simulink model "ensaios"  (R2012b)
settings: Solver=ode3  StartTime=0.0  StopTime=2  FixedStep=1e-4  RelTol=1e-6
libraries: BLDC x1
settings Model: BufferReuse=off  Creator=Juliano  LastModifiedBy=Juliano
settings DataIOCC: LimitDataPoints=off
settings OptimizationCC: OptimizeBlockIOStorage=off  BufferReuse=off  ExpressionFolding=off  LocalBlockOutputs=off

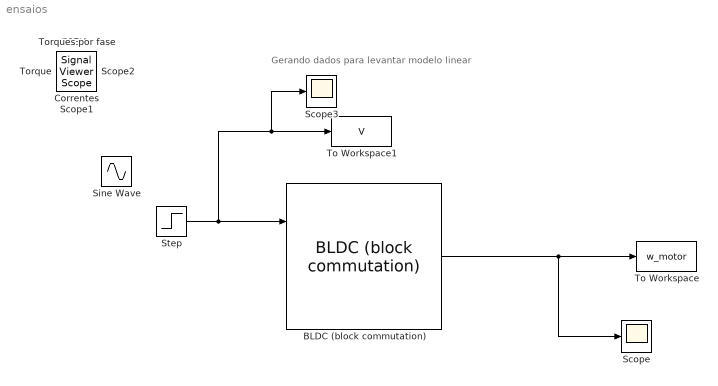
== system ensaios ==
  note: Gerando dados para levantar modelo linear
  BLDC (block commutation) : BLDC/BLDC (block commutation)  J=1.39e-6  R=10.1/2  L=2.04/2000  P=8  Kt=15.7e-3/1.19  Ke=15.7e-3/1.19  Kd=0
  Scope : Scope
  Scope3 : Scope
  Sine Wave : Sin  Amplitude=12  Frequency=10  SampleTime=0
  Step : Step  After=12  SampleTime=0
  To Workspace : ToWorkspace  VariableName=w_motor  SampleTime=-1
  To Workspace1 : ToWorkspace  VariableName=V  SampleTime=-1
  Correntes : SignalViewerScope  IOType=viewer  NumInputPorts=3  ZoomMode=yonly  RefreshTime=0.035000
      settings: YMin=-5~-5~-5  YMax=5~5~5
  FCEMs : SignalViewerScope  IOType=viewer  NumInputPorts=3  ZoomMode=xonly  RefreshTime=0.035000
      settings: YMin=-5~-5~-5  YMax=5~5~5  SaveName=ScopeData2
  Scope1 : SignalViewerScope  IOType=viewer  RefreshTime=0.035000
      settings: SaveName=ScopeData3
  Scope2 : SignalViewerScope  IOType=viewer  RefreshTime=0.035000
      settings: SaveName=ScopeData4
  Torque : SignalViewerScope  IOType=viewer  ZoomMode=xonly  RefreshTime=0.035000
      settings: SaveToWorkspace=on  SaveName=Torque
  Torques por fase : SignalViewerScope  IOType=viewer  NumInputPorts=3  ZoomMode=xonly  RefreshTime=0.035000
      settings: YMin=-5~-5~-5  YMax=5~5~5
  wires:
  Step/1 -> Scope3/1, To Workspace1/1, BLDC (block commutation)/1
  BLDC (block commutation)/2 -> Scope/1, To Workspace/1
